simulink model "jarmu"  (R2018b)
settings: Solver=VariableStepAuto  StartTime=0.0  StopTime=250  FixedStep=0.01  MaxStep=0.01  RelTol=1e-3
model workspace (MAT data in the model file):
  CdA = Simulink.Parameter
  CdA.Value = 0.576
  CdA.DataType = 'auto'
  CdA.Dimensions = [1 1]
  g = Simulink.Parameter
  g.Value = 9.81
  g.DataType = 'auto'
  g.Dimensions = [1 1]
  m = Simulink.Parameter
  m.Value = 2200
  m.DataType = 'auto'
  m.Dimensions = [1 1]
  p = Simulink.Parameter
  p.Value = 1.2
  p.DataType = 'auto'
  p.Dimensions = [1 1]
  v = Simulink.Parameter
  v.DataType = 'auto'
  v.Dimensions = [0 0]
undefined symbols (not defined in the file or in its folder): sigbuilder_block
libraries: simulink_extras x1
settings Model: Creator=cloud  LastModifiedBy=cloud
settings RTWCC: Description=Generic Real-Time Target  RTWCompilerOptimization=on
settings CodeAppCC: MaxIdLength=95

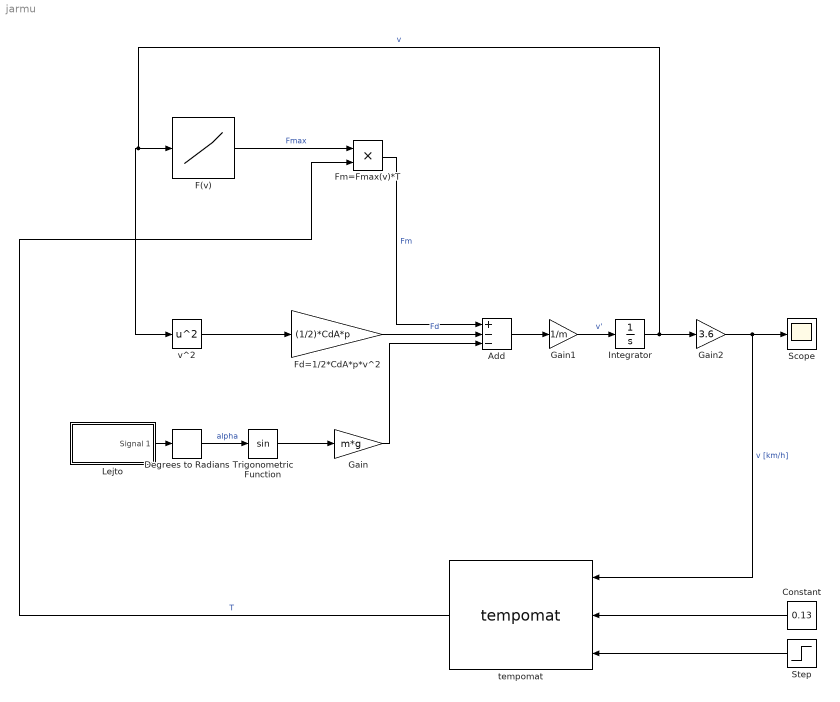
== system jarmu ==
  Add : Sum  Inputs=+--
  Constant : Constant  Value=0.13
  Degrees to Radians : simulink_extras/Transformations/Degrees to Radians
  F(v) : Lookup_n-D  NumberOfTableDimensions=1  BreakpointsForDimension1=[20 27 36 53]  Table=[14500 7200 3800 1900]  InterpMethod=Cubic spline  ExtrapMethod=Clip  InternalRulePriority=Speed  RndMeth=Simplest  InputSameDT=on
  Fd=1/2*CdA*p*v^2 : Gain  Gain=(1/2)*CdA*p
  Fm=Fmax(v)*T : Product
  Gain : Gain  Gain=m*g
  Gain1 : Gain  Gain=1/m
  Gain2 : Gain  Gain=3.6
  Integrator : Integrator  InitialCondition=37  LimitOutput=on  UpperSaturationLimit=100  LowerSaturationLimit=0
  Lejto : Subsystem  Tag=STV Subsys  LoadFcn=sigbuilder_block('load');  StartFcn=sigbuilder_block('start');  StopFcn=sigbuilder_block('stop');  ClipboardFcn=sigbuilder_block('clipboard');  mask(Sigbuilder block){tuvar=[0:10]}
      mask help: Simulink:masks:SigbuilderBlock_MD
      mask init:
      | if ~strcmp(get_param(bdroot(gcbh),'SimulationStatus'),'stopped') tuvar = sigbuilder_block('maskInit'); end
      settings: CopyFcn=sigbuilder_block('copy');  DeleteFcn=sigbuilder_block('delete');  ModelCloseFcn=sigbuilder_block('modelClose');  PreSaveFcn=sigbuilder_block('preSave');  PauseFcn=sigbuilder_block('pause');  ContinueFcn=sigbuilder_block('continue');  NameChangeFcn=sigbuilder_block('namechange');  OpenFcn=sigbuilder_block('open',[38.25 112.5 550.5 399.75 ]);  CloseFcn=sigbuilder_block('close');
      mask Display: plot(0, 0, 100, 100,[2, 2, 32, 32, 2], [68, 8, 8, 68, 68],[32, 2], [38, 38], [32, 19, 2],[53, 60, 44], [32, 17, 17, 2],[16, 16, 31, 31]);txt = getActiveGroup(gcbh);text(2, 100, txt,'verticalAlignment', 'top');
  Scope : Scope
  Step : Step  Time=10  SampleTime=0
  Trigonometric Function : Trigonometry
  tempomat : S-Function  InitFcn=try, set_param(gcb,'FunctionName','tempomat'), end  FunctionName=tempomat  Parameters=1,0.1  SFunctionModules=tempomat_wrapper  SFunctionDeploymentMode=off  EnableBusSupport=off  mask(S-Function Builder){}
      mask help: Simulink:masks:SFunctionBuilder_MD
      mask init:
      | val = [[.9  0.75 0.75 1 1 .9 .9 1]',[1 1 0.75 0.75 .9 .9 1 .9]'];try , sys = get_param(gcb,'SfunBuilderFcnName');if isempty(sys), sys = get_param(gcb,'FunctionName'); end,catch, sys = get_param(gcb,'FunctionName'); end
      settings: CopyFcn=set_param(gcbh,'LinkStatus','none')  PreSaveFcn=try, set_param(gcb,'FunctionName','tempomat'), end  OpenFcn=sfunctionwizard(gcbh)
      mask Display: plot(val(:,1),val(:,2)),disp(sys), port_label('input',1,'speed'), port_label('input',2,'pedal'), port_label('input',3,'onoff'), port_label('output',1,'output')
  v^2 : Math  Operator=square  SaturateOnIntegerOverflow=on
  wires:
  F(v)/1 -> Fm=Fmax(v)*T/1  "Fmax"
  tempomat/1 -> Fm=Fmax(v)*T/2  "T"
  Fm=Fmax(v)*T/1 -> Add/1  "Fm"
  Fd=1/2*CdA*p*v^2/1 -> Add/2  "Fd"
  v^2/1 -> Fd=1/2*CdA*p*v^2/1
  Trigonometric Function/1 -> Gain/1
  Degrees to Radians/1 -> Trigonometric Function/1  "alpha"
  Gain/1 -> Add/3
  Add/1 -> Gain1/1
  Gain1/1 -> Integrator/1  "v'"
  Integrator/1 -> v^2/1, F(v)/1, Gain2/1  "v"
  Gain2/1 -> tempomat/1, Scope/1  "v [km/h]"
  Constant/1 -> tempomat/2
  Step/1 -> tempomat/3
  Lejto/1(Signal 1) -> Degrees to Radians/1

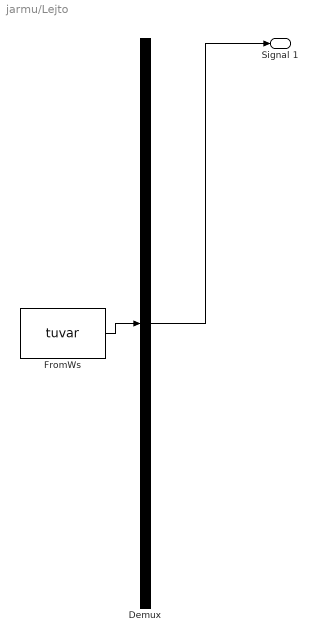
== system jarmu/Lejto ==
  Demux : Demux  Tag=STV Demux  Outputs=1
  FromWs : FromWorkspace  Tag=STV FromWs  VariableName=tuvar  SampleTime=0
      SigBuilderData=|
      | common.afterFinalStr = 'Extrapolate'
      | common.sampleTime = 0
      | dataSet.timeRange = [0 250]
      | dataSet.name = 'Group 1'
      | sbobj.Groups.Name = 'Group 1'
      | sbobj.Groups.Signals.Name = 'Signal 1'
      | sbobj.Groups.Signals.XData = [0 40 50 90 100 140 150 200 210 250]
      | sbobj.Groups.Signals.YData = [0 0 5 5 0 0 -1 -1 0 0]
      | sbobj.Groups.TimeRange = [0 250]
  Signal 1 : Outport  Tag=STV Outport
  wires:
  Demux/1 -> Signal 1/1
  FromWs/1 -> Demux/1
